simulink model "Longitudinal_acc_model"  (R2022b)
settings: Solver=VariableStepAuto  StartTime=0.0  StopTime=10.0  RelTol=1e-3
libraries: autolibshared x1, slpidlib x1
settings Model: Creator=Simon  LastModifiedBy=Simon

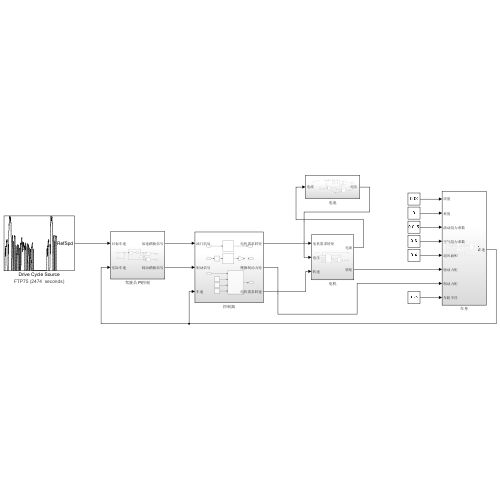
[thumbnail: Simulink's stored preview of the top-level diagram]
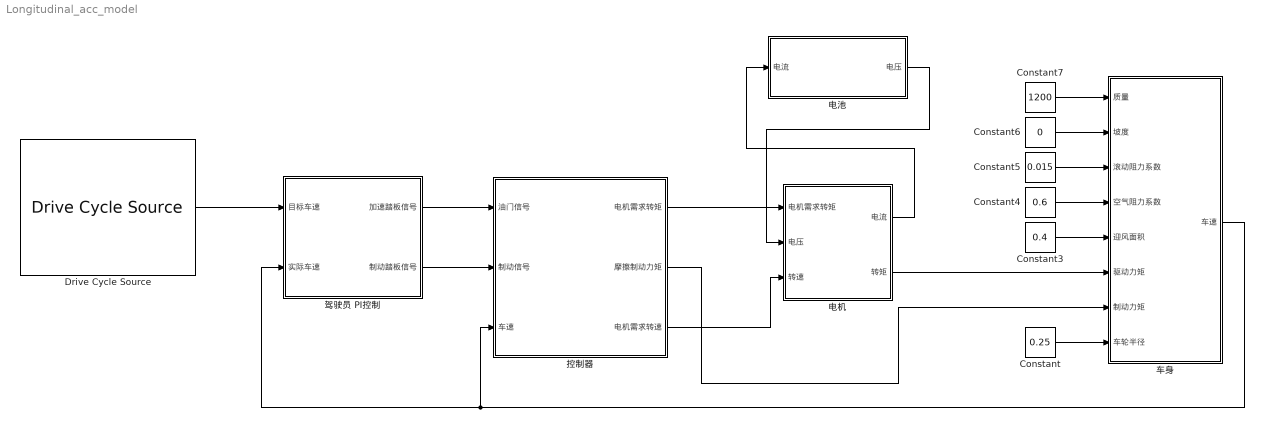
== system Longitudinal_acc_model ==
  Constant : Constant  Value=0.25
  Constant3 : Constant  Value=0.4
  Constant4 : Constant  Value=0.6
  Constant5 : Constant  Value=0.015
  Constant6 : Constant  Value=0
  Constant7 : Constant  Value=1200
  Drive Cycle Source : autolibshared/Drive Cycle Source  cycleVar=FTP75  fileVar=cycleFTP75.mat  tfinal="2474  seconds"  cycleRepeat=off  outAccPort=off  outGearPort=off  gearList=No gear data  t_wot1=5  xdot_woto=0  xdot_wot1=30  t_wot2=20  xdot_wot2=0  t_wotend=30  srcUnit=m/s  outUnit=km/h  srcAccUnit=m/s/s  outAccUnit=m/s^2  dt=0  aMode=1  faultOption=off  velBnd=2  velBndUnit=mph  inUnit=m/s  timeBnd=1  failOption=off  stopSim=off  maxFaultCnt=10  maxFaultTime=2  maxTotFaultTime=15  traceOption=off  dtTrace=1  traceWindow=10  lastDCname=FTP75  lastOutUnit=mph  lastDT=0  lastTB=1  lastSB=2  forceCalcBound=off
  控制器 : Subsystem
  电机 : Subsystem
  电池 : Subsystem
  车身 : Subsystem
  驾驶员 PI控制 : Subsystem
  wires:
  Constant/1 -> 车身/8(车轮半径)
  Constant6/1 -> 车身/2(坡度)
  Constant7/1 -> 车身/1(质量)
  Constant5/1 -> 车身/3(滚动阻力系数)
  Constant4/1 -> 车身/4(空气阻力系数)
  Constant3/1 -> 车身/5(迎风面积)
  控制器/2(摩擦制动力矩) -> 车身/7(制动力矩)
  控制器/1(电机需求转矩) -> 电机/1(电机需求转矩)
  控制器/3(电机需求转速) -> 电机/3(转速)
  电机/2(转矩) -> 车身/6(驱动力矩)
  电池/1("电压 ") -> 电机/2(电压)
  电机/1(电流) -> 电池/1(电流)
  驾驶员 PI控制/1(加速踏板信号) -> 控制器/1(油门信号)
  驾驶员 PI控制/2(制动踏板信号) -> 控制器/2(制动信号)
  车身/1(车速) -> 控制器/3(车速), 驾驶员 PI控制/2(实际车速)
  Drive Cycle Source/1 -> 驾驶员 PI控制/1(目标车速)

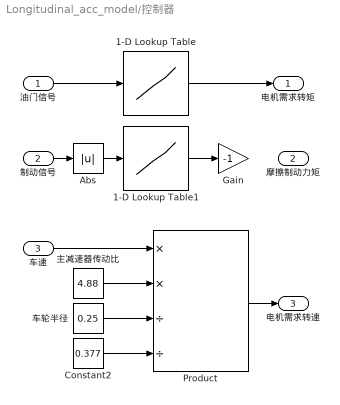
== system Longitudinal_acc_model/控制器 ==
  油门信号 : Inport
  制动信号 : Inport  Port=2
  车速 : Inport  Port=3
  1-D Lookup Table : Lookup_n-D  NumberOfTableDimensions=1  BreakpointsForDimension1=[0:1]  Table=[0 200]  InternalRulePriority=Speed  RndMeth=Simplest
  1-D Lookup Table1 : Lookup_n-D  NumberOfTableDimensions=1  BreakpointsForDimension1=[0:1]  Table=[0 3000]  InternalRulePriority=Speed  RndMeth=Simplest
  Abs : Abs  SaturateOnIntegerOverflow=off
  Constant2 : Constant  Value=0.377
  Gain : Gain  Gain=-1
  Product : Product  Inputs=**//
  主减速器传动比 : Constant  Value=4.88
  车轮半径 : Constant  Value=0.25
  电机需求转矩 : Outport
  摩擦制动力矩 : Outport  Port=2
  电机需求转速 : Outport  Port=3
  wires:
  油门信号/1 -> 1-D Lookup Table/1
  1-D Lookup Table/1 -> 电机需求转矩/1
  制动信号/1 -> Abs/1
  Abs/1 -> 1-D Lookup Table1/1
  1-D Lookup Table1/1 -> Gain/1
  车速/1 -> Product/1
  Constant2/1 -> Product/4
  车轮半径/1 -> Product/3
  主减速器传动比/1 -> Product/2
  Product/1 -> 电机需求转速/1

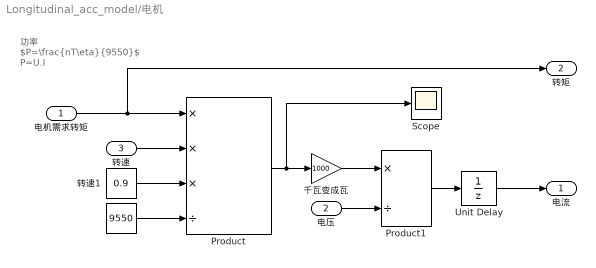
== system Longitudinal_acc_model/电机 ==
  note: 功率 $P=\frac{nT\eta}{9550}$
      | P=U.I
  电机需求转矩 : Inport
  电压 : Inport  Port=2
  转速 : Inport  Port=3
  " " : Constant  Value=9550
  Product : Product  Inputs=***/
  Product1 : Product  Inputs=*/
  Scope : Scope
  Unit Delay : UnitDelay  SampleTime=-1  HasFrameUpgradeWarning=on
  千瓦变成瓦 : Gain  Gain=1000
  转速1 : Constant  Value=0.9
  电流 : Outport
  转矩 : Outport  Port=2
  wires:
  电机需求转矩/1 -> 转矩/1, Product/1
  转速/1 -> Product/2
  " "/1 -> Product/4
  转速1/1 -> Product/3
  Product/1 -> Scope/1, 千瓦变成瓦/1
  千瓦变成瓦/1 -> Product1/1
  电压/1 -> Product1/2
  Product1/1 -> Unit Delay/1
  Unit Delay/1 -> 电流/1

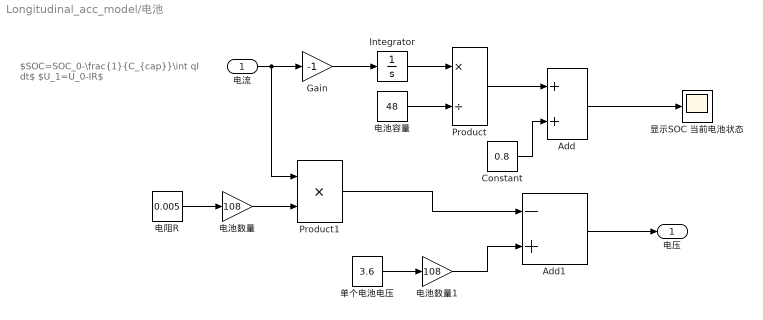
== system Longitudinal_acc_model/电池 ==
  note: $SOC=SOC_0-\frac{1}{C_{cap}}\int qI dt$
      | $U_1=U_0-IR$
  电流 : Inport
  Add : Sum
  Add1 : Sum  Inputs=-+
  Constant : Constant  Value=0.8
  Gain : Gain  Gain=-1
  Integrator : Integrator
  Product : Product  Inputs=*/
  Product1 : Product
  单个电池电压 : Constant  Value=3.6
  显示SOC 当前电池状态 : Scope
  电池容量 : Constant  Value=48
  电池数量 : Gain  Gain=108
  电池数量1 : Gain  Gain=108
  电阻R : Constant  Value=0.005
  "电压 " : Outport
  wires:
  Gain/1 -> Integrator/1
  电流/1 -> Product1/1, Gain/1
  电池容量/1 -> Product/2
  Integrator/1 -> Product/1
  Product/1 -> Add/1
  Constant/1 -> Add/2
  Add/1 -> 显示SOC 当前电池状态/1
  电阻R/1 -> 电池数量/1
  电池数量/1 -> Product1/2
  电池数量1/1 -> Add1/2
  单个电池电压/1 -> 电池数量1/1
  Product1/1 -> Add1/1
  Add1/1 -> "电压 "/1

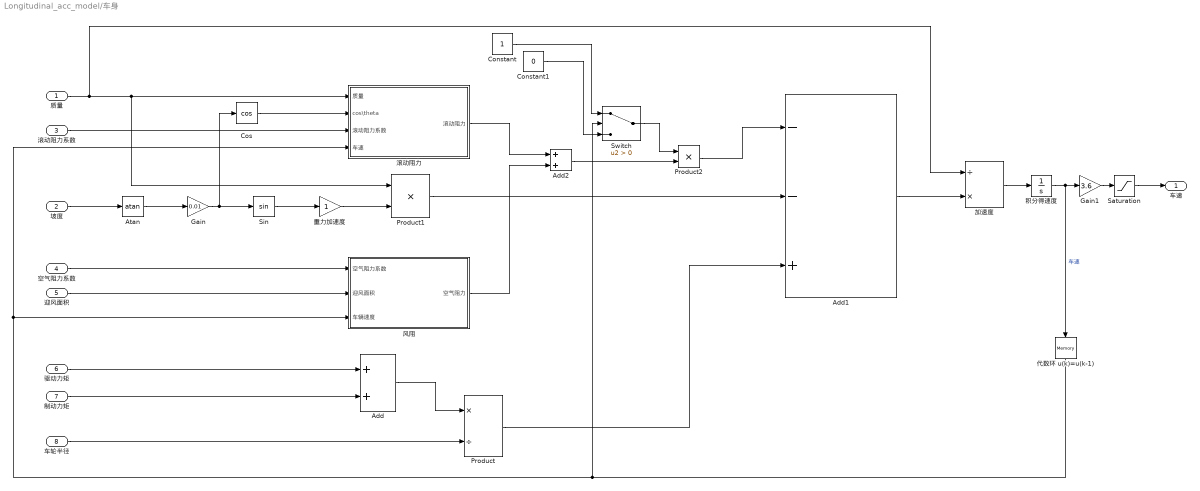
== system Longitudinal_acc_model/车身 ==
  质量 : Inport
  坡度 : Inport  Port=2
  滚动阻力系数 : Inport  Port=3
  空气阻力系数 : Inport  Port=4
  迎风面积 : Inport  Port=5
  驱动力矩 : Inport  Port=6
  制动力矩 : Inport  Port=7
  车轮半径 : Inport  Port=8
  Add : Sum
  Add1 : Sum  Inputs=--+
  Add2 : Sum
  Atan : Trigonometry  Operator=atan
  Constant : Constant
  Constant1 : Constant  Value=0
  Cos : Trigonometry  Operator=cos
  Gain : Gain  Gain=0.01
  Gain1 : Gain  Gain=3.6
  Product : Product  Inputs=*/
  Product1 : Product
  Product2 : Product
  Saturation : Saturate  UpperLimit=10000  LowerLimit=0
  Sin : Trigonometry
  Switch : Switch  Criteria=u2 > Threshold  SaturateOnIntegerOverflow=off  InputSameDT=off
  代数环 u(k)=u(k-1) : Memory
  加速度 : Product  Inputs=/*
  滚动阻力 : Subsystem
  积分得速度 : Integrator
  重力加速度 : Gain
  风阻 : Subsystem
  车速 : Outport
  wires:
  质量/1 -> 加速度/1, Product1/1, 滚动阻力/1(质量)
  空气阻力系数/1 -> 风阻/1(空气阻力系数)
  滚动阻力系数/1 -> 滚动阻力/3(滚动阻力系数)
  迎风面积/1 -> 风阻/2(迎风面积)
  驱动力矩/1 -> Add/1
  制动力矩/1 -> Add/2
  Add/1 -> Product/1
  车轮半径/1 -> Product/2
  坡度/1 -> Atan/1
  Atan/1 -> Gain/1
  Gain/1 -> Cos/1, Sin/1
  Cos/1 -> 滚动阻力/2(cos\theta)
  Sin/1 -> 重力加速度/1
  重力加速度/1 -> Product1/2
  积分得速度/1 -> 代数环 u(k)=u(k-1)/1, Gain1/1  "车速"
  Product/1 -> Add1/3
  Constant/1 -> Switch/1
  Constant1/1 -> Switch/3
  滚动阻力/1(滚动阻力) -> Add2/1
  风阻/1(空气阻力) -> Add2/2
  Add2/1 -> Product2/2
  Switch/1 -> Product2/1
  Product1/1 -> Add1/2
  Product2/1 -> Add1/1
  Add1/1 -> 加速度/2
  加速度/1 -> 积分得速度/1
  Gain1/1 -> Saturation/1
  Saturation/1 -> 车速/1
  代数环 u(k)=u(k-1)/1 -> 滚动阻力/4(车速), 风阻/3(车辆速度), Switch/2

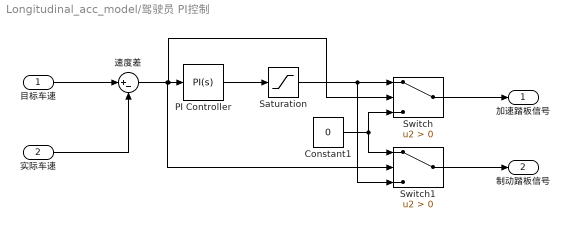
== system Longitudinal_acc_model/驾驶员 PI控制 ==
  目标车速 : Inport
  实际车速 : Inport  Port=2
  Constant1 : Constant  Value=0
  PI Controller : slpidlib/PID Controller  Controller=PI  Form=Parallel  TimeDomain=Continuous-time  UseExternalTs=off  SampleTime=-1  IntegratorMethod=Forward Euler  FilterMethod=Forward Euler  ControllerParametersSource=internal  P=1  I=1  UseKiTs=off  D=0  N=100  UseFilter=on  TunerSelectOption=Transfer Function Based (PID Tuner App)  InitialConditionSource=internal  InitialConditionForIntegrator=0  InitialConditionForFilter=0  DifferentiatorICPrevScaledInput=0  ExternalReset=none  TrackingMode=off  Kt=1  LimitOutput=off  SatLimitsSource=internal  UpperSaturationLimit=inf  LowerSaturationLimit=-inf  LinearizeAsGain=on  AntiWindupMode=none  Kb=1  LimitIntegrator=off  UpperIntegratorSaturationLimit=inf  LowerIntegratorSaturationLimit=-inf  POutMin=[]  POutMax=[]  IOutMin=[]  IOutMax=[]  DOutMin=[]  DOutMax=[]  NOutMin=[]  NOutMax=[]  SumOutMin=[]  SumOutMax=[]  SaturationOutMin=[]  SaturationOutMax=[]  PParamMin=[]  PParamMax=[]  IParamMin=[]  IParamMax=[]  DParamMin=[]  DParamMax=[]  NParamMin=[]  NParamMax=[]  KbParamMin=[]  KbParamMax=[]  KtParamMin=[]  KtParamMax=[]  KbOutMin=[]  KbOutMax=[]  KtOutMin=[]  KtOutMax=[]  IntegratorOutMin=[]  IntegratorOutMax=[]  FilterOutMin=[]  FilterOutMax=[]  SumI1OutMin=[]  SumI1OutMax=[]  SumI2OutMin=[]  SumI2OutMax=[]  SumI3OutMin=[]  SumI3OutMax=[]  SumI4OutMin=[]  SumI4OutMax=[]  SumDOutMin=[]  SumDOutMax=[]  DifferentiatorOutMin=[]  DifferentiatorOutMax=[]  FilterDiffOutCoefMin=[]  FilterDiffOutCoefMax=[]  ReciprocalOutMin=[]  ReciprocalOutMax=[]  SumDenOutMin=[]  SumDenOutMax=[]  SumNumOutMin=[]  SumNumOutMax=[]  DivideOutMin=[]  DivideOutMax=[]  UdiffTsProdOutMin=[]  UdiffTsProdOutMax=[]  NTsProdOutMin=[]  NTsProdOutMax=[]  UintegralTsProdOutMin=[]  UintegralTsProdOutMax=[]  UngainTsProdOutMin=[]  UngainTsProdOutMax=[]  ClampingZeroOutDataTypeStr=Inherit: Inherit via back propagation  ClampingZeroOutMin=[]  ClampingZeroOutMax=[]  FilterDenConstantOutDataTypeStr=Inherit: Inherit via back propagation  FilterDenConstantOutMin=[]  FilterDenConstantOutMax=[]  PCopyOutDataTypeStr=Inherit: Inherit via back propagation  PCopyOutMin=[]  PCopyOutMax=[]  NCopyOutDataTypeStr=Inherit: Inherit via back propagation  NCopyOutMin=[]  NCopyOutMax=[]  IntegratorContinuousStateAttributes=''  IntegratorStateMustResolveToSignalObject=off  IntegratorRTWStateStorageClass=Auto  FilterContinuousStateAttributes=''  FilterStateMustResolveToSignalObject=off  FilterRTWStateStorageClass=Auto  ParallelPVariant=InternalParameters  IdealPVariant=Disabled  IVariant=InternalParameters  DVariant=Disabled  IntegratorVariant=Continuous  SatVariant=Disabled  AWVariant=Passthrough  PCopyVariant=Disabled  TRVariant=Disabled  FdbkBlocksVariant=Forward  IdealPFdbkVariant=Disabled  SatFdbkVariant=Disabled  DerivativeFilterVariant=Disabled  NVariant=Disabled  NCopyVariant=Disabled_SignalSpec  FilterICVariant=Disabled  IntegratorICVariant=InternalICs  ExternalResetVariant=Disabled  TRSumVariant=Passthrough  SumFdbkVariant=Disabled  SumVariant=Sum_PI  TsampFilterVariant=InternalTs  TsampNgainVariant=Passthrough  TsampIntegralVariant=Passthrough  ExternalSaturationOutDataTypeStr=Inherit: Same as second input
  Saturation : Saturate  UpperLimit=1  LowerLimit=-1
  Switch : Switch  Criteria=u2 > Threshold  SaturateOnIntegerOverflow=off  InputSameDT=off
  Switch1 : Switch  Criteria=u2 > Threshold  SaturateOnIntegerOverflow=off  InputSameDT=off
  速度差 : Sum  Inputs=|+-
  加速踏板信号 : Outport
  制动踏板信号 : Outport  Port=2
  wires:
  目标车速/1 -> 速度差/1
  实际车速/1 -> 速度差/2
  速度差/1 -> Switch1/2, Switch/2, PI Controller/1
  PI Controller/1 -> Saturation/1
  Saturation/1 -> Switch1/3, Switch/1
  Constant1/1 -> Switch1/1, Switch/3
  Switch/1 -> 加速踏板信号/1
  Switch1/1 -> 制动踏板信号/1

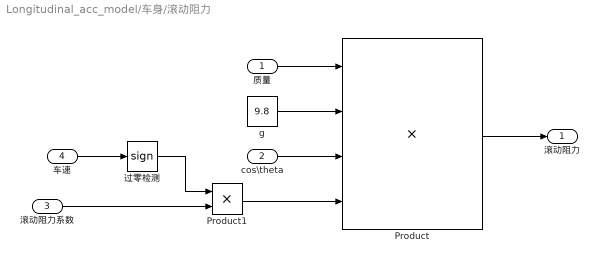
== system Longitudinal_acc_model/车身/滚动阻力 ==
  质量 : Inport
  cos\theta : Inport  Port=2
  滚动阻力系数 : Inport  Port=3
  车速 : Inport  Port=4
  Product : Product  Inputs=4
  Product1 : Product
  g : Constant  Value=9.8
  过零检测 : Signum
  滚动阻力 : Outport
  wires:
  质量/1 -> Product/1
  g/1 -> Product/2
  cos\theta/1 -> Product/3
  Product/1 -> 滚动阻力/1
  滚动阻力系数/1 -> Product1/2
  Product1/1 -> Product/4
  车速/1 -> 过零检测/1
  过零检测/1 -> Product1/1

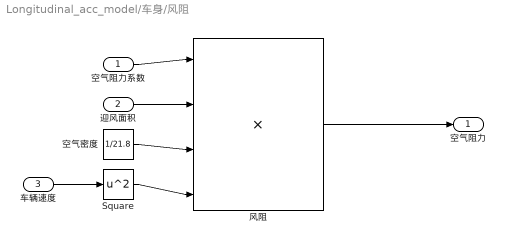
== system Longitudinal_acc_model/车身/风阻 ==
  空气阻力系数 : Inport
  迎风面积 : Inport  Port=2
  车辆速度 : Inport  Port=3
  Square : Math  Operator=square
  空气密度 : Constant  Value=1/21.8
  风阻 : Product  Inputs=4
  空气阻力 : Outport
  wires:
  风阻/1 -> 空气阻力/1
  空气阻力系数/1 -> 风阻/1
  车辆速度/1 -> Square/1
  Square/1 -> 风阻/4
  空气密度/1 -> 风阻/3
  迎风面积/1 -> 风阻/2
